simulink model "lab9"  (R2024a)
settings: Solver=VariableStepAuto  StartTime=0.0  StopTime=10.0  RelTol=1e-3
values from neighbouring files (symbols this model uses):
  m = 5    [lab3_1.m]    (also in lab43_2.m = 200)
  n = 7    [lab3_1.m]    (also in test.m = length(polynomial1_bin); test_OCMC.m = length(seq1))
libraries: simulink x2, matrix_library x1
settings Model: Creator=QQshnik  LastModifiedBy=QQshnik

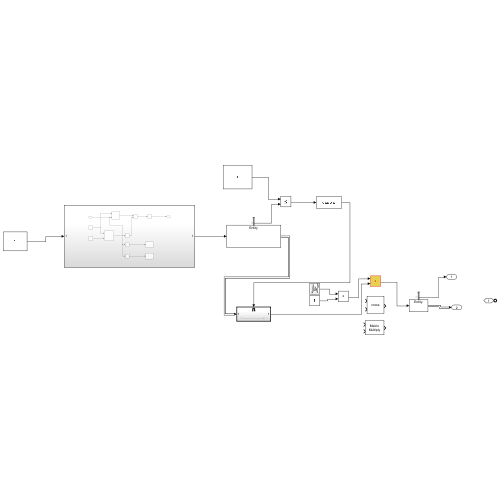
[thumbnail: Simulink's stored preview of the top-level diagram]
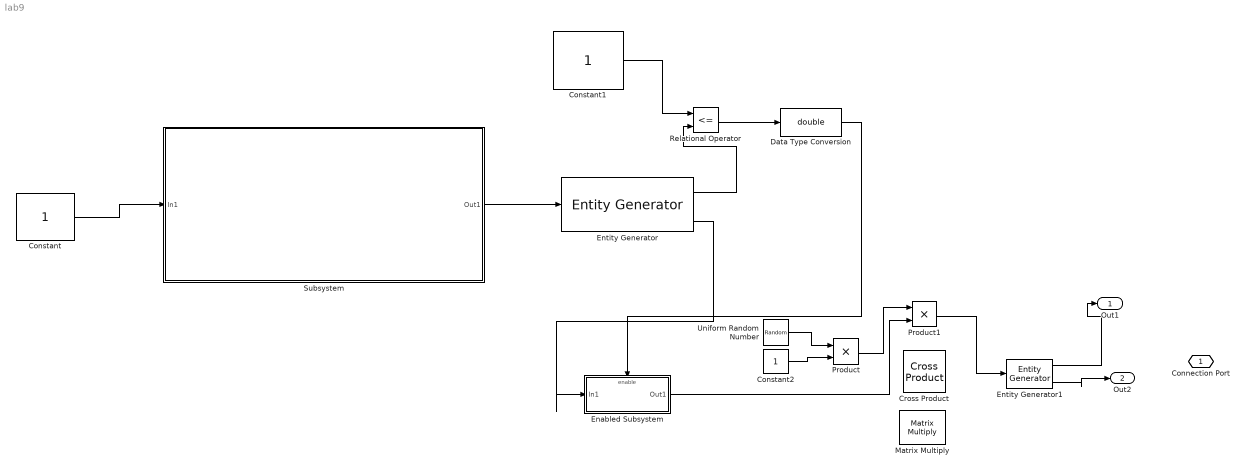
== system lab9 ==
  Constant : Constant
  Constant1 : Constant
  Constant2 : Constant
  Cross Product : matrix_library/Cross Product
  Data Type Conversion : DataTypeConversion  OutDataTypeStr=double  SaturateOnIntegerOverflow=off  RndMeth=Floor
  Enabled Subsystem : Subsystem  TreatAsAtomicUnit=on
  Entity Generator : EntityGenerator  OutputPortMessageModes=n,m  TimeSource=Signal port  NumberEntitiesDeparted=on  EntityType=Structured  EntityTypeName=Entity
      settings: InputPortMap=u1  OutputPortMap=o0,o3
  Entity Generator1 : EntityGenerator  OutputPortMessageModes=n,m  TimeSource=Signal port  NumberEntitiesDeparted=on  EntityType=Structured  EntityTypeName=Entity
      settings: InputPortMap=u1  OutputPortMap=o0,o3
  Matrix Multiply : Product  Multiplication=Matrix(*)
  Product : Product
  Product1 : Product
  Relational Operator : RelationalOperator  Operator=<=  OutDataTypeStr=boolean  RndMeth=Simplest  InputSameDT=off
  Subsystem : Subsystem
  Uniform Random Number : UniformRandomNumber  SampleTime=0.1
  Connection Port : PMIOPort  Side=Left
  Out1 : Outport
  Out2 : Outport  Port=2
  wires:
  Subsystem/1(Out1) -> Entity Generator/1
  Constant/1 -> Subsystem/1(In1)
  Entity Generator/1 -> Relational Operator/2
  Constant1/1 -> Relational Operator/1
  Entity Generator/2 -> Enabled Subsystem/1(In1)
  Relational Operator/1 -> Data Type Conversion/1
  Data Type Conversion/1 -> Enabled Subsystem/Enable
  Uniform Random Number/1 -> Product/1
  Constant2/1 -> Product/2
  Enabled Subsystem/1(Out1) -> Product1/2
  Product/1 -> Product1/1
  Entity Generator1/1 -> Out1/1
  Product1/1 -> Entity Generator1/1
  Entity Generator1/2 -> Out2/1

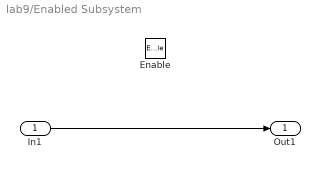
== system lab9/Enabled Subsystem ==
  In1 : Inport
  Enable : EnablePort
  Out1 : Outport
  wires:
  In1/1 -> Out1/1

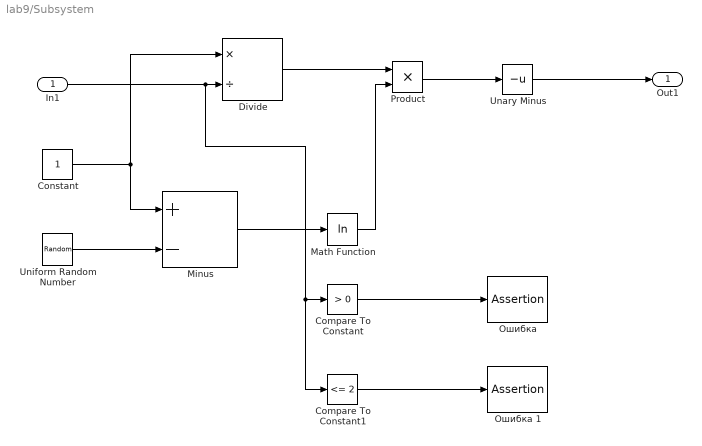
== system lab9/Subsystem ==
  In1 : Inport
  Compare To Constant : simulink/Logic and Bit Operations/Compare To Constant  relop=>  const=0  OutDataTypeStr=boolean
  Compare To Constant1 : simulink/Logic and Bit Operations/Compare To Constant  relop=<=  const=2  OutDataTypeStr=boolean
  Constant : Constant
  Divide : Product  Inputs=*/
  Math Function : Math  Operator=log
  Minus : Sum  Inputs=+-
  Product : Product
  Unary Minus : UnaryMinus
  Uniform Random Number : UniformRandomNumber  SampleTime=0.1
  Ошибка : Assertion
  Ошибка 1 : Assertion
  Out1 : Outport
  wires:
  Constant/1 -> Divide/1, Minus/1
  In1/1 -> Compare To Constant1/1, Compare To Constant/1, Divide/2
  Math Function/1 -> Product/2
  Uniform Random Number/1 -> Minus/2
  Minus/1 -> Math Function/1
  Compare To Constant/1 -> Ошибка/1
  Divide/1 -> Product/1
  Compare To Constant1/1 -> Ошибка 1/1
  Product/1 -> Unary Minus/1
  Unary Minus/1 -> Out1/1
